simulink model "sim_all"  (R2020a)
settings: Solver=VariableStepAuto  StartTime=0.0  StopTime=2000  RelTol=1e-3
undefined symbols (not defined in the file or in its folder): a1, a2, alpha1, alpha2, cornerA, cornerB, cornerC, cornerD, ctrl_clockwise, ctrl_int_bound_or, ctrl_int_bound_pos, ctrl_k_or, ctrl_k_pos, ctrl_Ki_vel, ctrl_Kp_v_pos, ctrl_Kp_vel, ctrl_TAM, ctrl_Ts, ctrl_va_uncontrolled, ctrl_vel_uncontrolled, D, dead_zone_limit, depth, DiscIntNeverNeededParam, distanceFromWall, initInspectedSide, initPoint, mod_A, mod_Cd_F, mod_Cd_M, mod_eta_init, mod_g, mod_h0, mod_Ixx, mod_Iyy, mod_Izz, mod_Kp_dot, mod_lat0, mod_lon0, mod_m, mod_Mq_dot, mod_ni_init, mod_Nr_dot, mod_p1, mod_p2, mod_p3, mod_p4, mod_p5, mod_p6, mod_R, mod_Rm, mod_t1, mod_t2, mod_t3, mod_t4, mod_t5, mod_t6, mod_W, mod_Xu_dot, mod_Yv_dot ... (+53)
libraries: simulink x8, cstblocks x6, simulink_extras x1
(part 4 of 6)

== matlab function sim_all/Mission_supervisor_v3/Mission_Supervisor/Orientazione in profondità/MATLAB Function ==
  data: delta_current_or_prof output; delta_stato_or_prof output; Pos_d output size=3; Dpp_d output; Orp_d output; Pos_s input; Orp_s input; relativeDirection parameter; depth parameter; punto_iniz_patt input; error_flag input; soglia_orp parameter; soglia_SOS_pos parameter; SOS parameter; distanceFromWall parameter
function [delta_current_or_prof, delta_stato_or_prof, Pos_d, Dpp_d, Orp_d] = Orientazione_profondita(Pos_s, Orp_s, relativeDirection, depth, punto_iniz_patt, error_flag, soglia_orp, soglia_SOS_pos, SOS, distanceFromWall)

    disp("Orientazione in profondita");
    
    %% Unità di misura 
    
    % Pos_d, Pos_s, punto_iniz_patt, soglia_SOS_pos                        [deg, deg, m]
    % Orp_d, Orp_s, soglia_orp                                             [rad]
    % relativeDirection                                                    [deg]
    % Dpp_d, depth, distanceFromWall                                       [m]

    %% Inizializzazione variabili
    
    % Utilizzata per la permanenza nello stato corrente
    delta_stato_or_prof = 0;
    
    pronti = false;

    %% Preparazione dei riferimenti da fornire ai blocchi successivi
                
    % Posizione da mantenere
    Pos_d = [punto_iniz_patt(1); punto_iniz_patt(2); depth];
                                                                            %*****TEST******%
                                                                            %Pos_d = [43; 11; 0];
    
  
    % Orientazione da raggiungere
    Orp_d = deg2rad(relativeDirection);
    
    % Distanza dalla parete da mantenere
    Dpp_d = distanceFromWall;
    
    
    % Transizione di stato effettiva
    delta_current_or_prof = 104 - 103; 
    
    
    %% Verifiche
    
    % Verifica della corretta posizione
    if (abs(Pos_s(1) - Pos_d(1)) > soglia_SOS_pos(1) || ...
        abs(Pos_s(2) - Pos_d(2)) > soglia_SOS_pos(2) || ...
        abs(Pos_s(3) - Pos_d(3)) > soglia_SOS_pos(3))
    
        SOS = 1;
        disp("EMERGENZA:");
        
        if (abs(Pos_s(1) - Pos_d(1)) > soglia_SOS_pos(1))
            disp("Rilevato errore sulla posizione X");
        end
        if (abs(Pos_s(2) - Pos_d(2)) > soglia_SOS_pos(2))
            disp("Rilevato errore sulla posizione Y");
        end
        if (abs(Pos_s(3) - Pos_d(3)) > soglia_SOS_pos(3))
            disp("Rilevato errore sulla profondita Z");
        end
        
    end
    
    if error_flag == 1
        disp("EMERGENZA: errore segnalato dagli altri sottosistemi");
        SOS = 1;
    end
     
    % Si verifica di aver raggiunto l'orientazione desiderata
    if (SOS == 0 && ...
        abs(Orp_s - Orp_d) < soglia_orp)
    
        pronti = true;
    end
    
    %% Decisione dello stato successivo
    
    if pronti == true
        
        delta_stato_or_prof = 201 - 104; % Transizione eseguita correttamente
    end
    if SOS == 1
            
            delta_stato_or_prof = 301 - 104; % Transizione nello stato di emergenza
    end
    
    % Si rimane nello stato corrente
    

end

== matlab function sim_all/Mission_supervisor_v3/Mission_Supervisor/Frenata pattugliamento/MATLAB Function ==
  data: delta_current_fren_patt output; delta_stato_fren_patt output; contatore input; Pos_d output size=3; Dpp_d output; Dps_d output; Orp_d output; Pos_s input; Dpp_s input; Dps_s input; Orp_s input; distanceFromWall parameter; relativeDirection parameter; depth parameter; error_flag input; soglia_SOS_orp parameter; soglia_SOS_pos parameter; soglia_SOS_parete parameter; SOS parameter; soglia_parete parameter
function [delta_current_fren_patt, delta_stato_fren_patt, Pos_d, Dpp_d, Dps_d, Orp_d] = Frenata_pattugliamento(contatore, Pos_s, Dpp_s, Dps_s, Orp_s, distanceFromWall, relativeDirection, depth, error_flag, soglia_SOS_orp, soglia_SOS_pos, soglia_SOS_parete, SOS,soglia_parete)

    disp("Frenata (durante il pattugliamento)");
    
    %% Unità di misura 
    
    % Pos_d, Pos_s, soglia_SOS_pos                                                                 [deg, deg, m]
    % Orp_d, Orp_s, soglia_SOS_orp                                                                 [rad]
    % relativeDirection                                                                            [deg]
    % Dpp_d, Dps_d, Dpp_s, Dps_s, distanceFromWall, depth, soglia_SOS_parete, soglia_parete        [m]

    %% Inizializzazione variabili
   
    % Utilizzata per permanere nello stato corrente
    delta_stato_fren_patt = contatore;
    
    pronti = false;
    
    %% Preparazione dei riferimenti da fornire ai blocchi successivi
    
    % Profondità da mantenere
    Pos_d = [nan; nan; depth];
                                                                            %*****TEST******%
                                                                            %Pos_d = [nan; nan; 0];
    
    % Distanza dalla parete da mantenere
    Dpp_d = distanceFromWall;
    Dps_d = distanceFromWall;
    
    % Orientazione da mantenere
    Orp_d = deg2rad(relativeDirection);
    
    % Transizione di stato effettiva
    delta_current_fren_patt = 202 - 201 + contatore;  
    
    
    %% Verifiche
    
    % Verifica sulla corretta orientazione, profondità e distanza dalla parete pattugliata
    if (abs(Orp_s - Orp_d) > soglia_SOS_orp || ...
        abs(Dpp_s - Dpp_d) > soglia_SOS_parete || ...
        abs(Pos_s(3) - Pos_d(3)) > soglia_SOS_pos(3))
    
        SOS = 1;
        disp("EMERGENZA:");
        
        if (abs(Orp_s - Orp_d) > soglia_SOS_orp)
            disp("Rilevato errore sull'orientazione relativa");
        end
        
        if (abs(Dpp_s - Dpp_d) > soglia_SOS_parete)
            disp("Rilevato errore sulla distanza da parete");
        end
        
        if (abs(Pos_s(3) - Pos_d(3)) > soglia_SOS_pos(3))
            disp("Rilevato errore sulla profondita Z");
        end
        
    end
    
    if error_flag == 1
        disp("EMERGENZA: errore segnalato dagli altri sottosistemi");
        SOS = 1;
    end
     
                                                                            %*****TEST******%
                                                                            %test=0;
                                                                            %Serve per testare di rimanere 
                                                                            %in attesa in questo stato
                                                                            % if(contatore>2)
                                                                            %    test=100;
                                                                            % else
                                                                            %    test=0;
                                                                            % end

    % Si verifica di aver raggiunto la posizione desiderata in termini di 
    % distanza dalla parete successiva
    if (SOS == 0 && ...
        abs(Dps_s - Dps_d) < soglia_parete)
    
        pronti = true;
        
    end

    %% Decisione dello stato successivo
    
    if pronti == true
        
        delta_stato_fren_patt = 203 - 202 + contatore; % Transizione eseguita correttamente
    end
    if SOS == 1
            
            delta_stato_fren_patt = 301 - 202 + contatore; % Transizione nello stato di emergenza
    end
    % Si rimane nello stato corrente

end

== matlab function sim_all/Mission_supervisor_v3/Mission_Supervisor/Manovra/MATLAB Function ==
  data: delta_current_man output; delta_stato_man output; contatore output; contatore input; Pos_d output size=3; Dpp_d output; Dps_d output; Orp_d output; Pos_s input; Dpp_s input; Orp_s input; distanceFromWall parameter; relativeDirection parameter; depth parameter; error_flag input; soglia_orp parameter; soglia_SOS_parete parameter; soglia_SOS_pos parameter; SOS parameter; Dps_s input; alfa input; giro input; parete_attuale input
function [delta_current_man, delta_stato_man, contatore, Pos_d, Dpp_d, Dps_d, Orp_d] = Manovra(contatore, Pos_s, Dpp_s, Orp_s, distanceFromWall, relativeDirection, depth, error_flag, soglia_orp, soglia_SOS_parete, soglia_SOS_pos, SOS, Dps_s, alfa, giro, parete_attuale)

    disp("Manovra");
    
    %% Unità di misura 
     
    % Pos_d, Pos_s, soglia_SOS_pos                                                [deg,deg,m]
    % Orp_d, Orp_s, soglia_orp, alfa                                              [rad]
    % relativeDirection                                                           [deg]
    % Dpp_d, Dps_d, Dpp_s, Dps_s, distanceFromWall, depth, soglia_SOS_parete      [m]


    %% Inizializzazione variabili
    
    delta_stato_man = -2 * contatore;
    
    pronti = false;
    
    relativeDirection_rad = deg2rad(relativeDirection);
    
    % Si utilizza la variabile booleana giro, inizializzata nella matlab function "aggiornamento della parete"
    % per determinare il senso di pattugliamento
    if giro == 0 % orario
        inspectionDirection = "clockwise";
    else % antiorario
        inspectionDirection = "counterclockwise";
    end

    %% Preparazione dei riferimenti da fornire si blocchi successivi
          
    Pos_d = [nan; nan; depth];
                                                                            %*****TEST******%
                                                                            %Pos_d = [nan; nan; 0];
    % Distanza dalla parete da mantenere
    Dpp_d = distanceFromWall;
    Dps_d = distanceFromWall;
    
    % Orientazione relativa alla parete
    Orp_d = relativeDirection_rad;
    
    % In questo stato il riferimento di orientazione passato al controllo
    % si riferisce alla parete successiva. Questo rende necessario
    % l'introduzione della variabile "Orp_rif" utilizzata nelle condizioni
    % di switch poiché il valore di stima si riferisce ancora alla parete attuale.
    % I valori alfa corrispondono agli angoli interni ai corner del bacino.
    if (strcmp(inspectionDirection,'clockwise') == 1) % AB-BC-CD-DA
        
        if parete_attuale == 1 % pattugliamento AB, manovra in B
            Orp_rif = relativeDirection_rad + alfa(2); 
        elseif parete_attuale == 2 % pattugliamento BC, manovra in C
            Orp_rif = relativeDirection_rad + alfa(3);
        elseif parete_attuale == 3 % pattugliamento CD, manovra in D
            Orp_rif = relativeDirection_rad + alfa(4);
        else  % pattugliamento DA, manovra in A
            Orp_rif = relativeDirection_rad + alfa(1);
        end
        
    else % AB-DA-CD-BC
        
        if parete_attuale == 1 % pattugliamento AB, manovra in A
            Orp_rif = relativeDirection_rad - alfa(1);
        elseif parete_attuale == 2 % pattugliamento BC, manovra in B
            Orp_rif = relativeDirection_rad - alfa(2);
        elseif parete_attuale == 3 % pattugliamento CD, manovra in C
            Orp_rif = relativeDirection_rad - alfa(3);
        else % pattugliamento DA, manovra in D
            Orp_rif = relativeDirection_rad - alfa(4);
        end
    end
      
    % Transizione di stato effettiva
    delta_current_man = 203 - 202 + contatore;           
    
       
    %% Verifiche
    
    % Verifica di aver mantenuto la corretta profondità e distanza
    % dalle pareti considerate
    if (abs(Pos_s(3) - Pos_d(3)) > soglia_SOS_pos(3) || ...
       abs(Dpp_s - Dpp_d) > soglia_SOS_parete || ...
       abs(Dps_s - Dps_d) > soglia_SOS_parete)
    
        SOS = 1;
        disp("EMERGENZA:");
        
        if (abs(Pos_s(3) - Pos_d(3)) > soglia_SOS_pos(3))
            disp("Rilevato errore sulla profondita");
        end
        if (abs(Dpp_s - Dpp_d) > soglia_SOS_parete)
            disp("Rilevato errore sulla distanza da parete");
        end
        if (abs(Dps_s - Dps_d) > soglia_SOS_parete)
            disp("Rilevato errore sulla distanza da parete successiva");
        end
    end
    
                                                                            %*****TEST******%
                                                                            % if(contatore > 1)
                                                                            %     error_flag = 1;
                                                                            % end

     if error_flag == 1
        disp("EMERGENZA: errore segnalato dagli altri sottosistemi");
        SOS = 1;
     end
     
     
                                                                            %*****TEST******%
                                                                            %Serve per testare di rimanere 
                                                                            %in attesa in questo stato 
                                                                            %test = 0;
                                                                            %if(contatore > 2)%test
                                                                            %    test = 100;
                                                                            %else
                                                                            %    test = 0;
                                                                            %end
                                                                            
    % Si verifica di aver raggiunto l'orientazione desiderata 
    if (SOS == 0 && ...
        abs(Orp_s - Orp_rif) < soglia_orp)    
    
        pronti = true;
        
    end
    
    % La parete viene aggiornata soltanto
    % al termine della fase di manovra incrementando il contatore
    if pronti == true
         contatore = contatore + 1;
    end
    
     
    %% Decisione dello stato successivo
    
    if pronti == true
        if contatore < 4    % Non è ancora il pattugliamento dell'ultima parete 
            
            delta_stato_man = 201 - 203 - 2 * contatore +2;   % Si continua il pattugliamento delle pareti successive  
            
        else    % Completato il pattugliamento dell'ultima parete intera, si esce dal ciclo per
                % effettuare il pattugliamento parziale della parete
                % iniziale che era stata pattugliata solo per metà
                
            delta_stato_man = 204-203 - 2 * contatore +2;         
        end
    end
    
    if SOS == 1
            
            delta_stato_man = 301-203 + - 2 * contatore; %Transizione nello stato di emergenza
    end
        % Si rimane nello stato corrente

end

== matlab function sim_all/Mission_supervisor_v3/Mission_Supervisor/Completamento/MATLAB Function ==
  data: delta_current_comp output; parete input; delta_stato_comp output; Pos_d output size=3; Vel_d output; Dpp_d output; Orp_d output; Pos_s input; Vel_s input; Dpp_s input; Dps_s input; Orp_s input; depth parameter; speed parameter; distanceFromWall parameter; relativeDirection parameter; dps_fin input; error_flag input; soglia_SOS_vel parameter; soglia_parete_frenata parameter; soglia_SOS_orp parameter; soglia_SOS_pos parameter; soglia_SOS_parete parameter; SOS parameter; giro input
function [delta_current_comp, delta_stato_comp, Pos_d, Vel_d, Dpp_d, Orp_d] = Completamento(parete, Pos_s, Vel_s, Dpp_s, Dps_s, Orp_s, depth, speed, distanceFromWall, relativeDirection, dps_fin, error_flag, soglia_SOS_vel, soglia_parete_frenata, soglia_SOS_orp, soglia_SOS_pos, soglia_SOS_parete, SOS, giro)

    disp("Completamento del pattugliamento parziale della parete " + parete);
    
    %% Unità di misura 
    
    % Pos_d, Pos_s, soglia_SOS_pos                                                                              [deg, deg, m]
    % Orp_d, Orp_s, soglia_SOS_orp                                                                              [rad]
    % relativeDirection                                                                                         [deg]
    % Dpp_d, Dps_d, Dpp_s, Dps_s, dps_fin, distanceFromWall, depth, soglia_SOS_parete, soglia_parete_frenata    [m]
    % Vel_d, Vel_s, speed, soglia_SOS_vel                                                                       [m/s]

    %% Inizializzazione variabili
    
    % Utilizzata per permanere in questo stato e inizializzata a zero
    % perché fuori dal ciclo
    delta_stato_comp = 0; 
    
    pronti = false;
    
    
    %% Preparazione dei riferimenti da fornire ai blocchi successivi
    
    % Profondità da mantenere
    Pos_d = [nan; nan; depth];
                                                                            %*****TEST******%
                                                                            %Pos_d = [nan; nan; 0];
    
    % Velocità da raggiungere
    Vel_d = speed;              
                                                                            %*****TEST******%
                                                                            %Vel_d_vett = [0; 0; 0];

    % Distanza dalla parete da mantenere
    Dpp_d = distanceFromWall;
    
    % Orientazione da mantenere
    Orp_d = deg2rad(relativeDirection);
        
    % Transizione di stato effettiva
    delta_current_comp = 204 - 203;  
  
    %% Verifiche
    
    % Verifica sulla corretta profondità, orientazione, distanza dalla parete pattugliata 
    % e velocità
    if (abs(Pos_s(3) - Pos_d(3)) > soglia_SOS_pos(3) || ...
        abs(Orp_s - Orp_d) > soglia_SOS_orp || ...
        abs(Dpp_s - Dpp_d) > soglia_SOS_parete || ...
        norm(Vel_s) - Vel_d > soglia_SOS_vel)
    
        SOS = 1;
        disp("EMERGENZA:");
        
        if (abs(Orp_s - Orp_d) > soglia_SOS_orp)
            disp("Rilevato errore sull'orientazione relativa");
        end
        
        if (abs(Dpp_s - Dpp_d) > soglia_SOS_parete)
            disp("Rilevato errore sulla distanza da parete");
        end
        
        if (abs(Pos_s(3) - Pos_d(3)) > soglia_SOS_pos(3))
            disp("Rilevato errore sulla profondita Z");
        end
        
        if (norm(Vel_s) - Vel_d > soglia_SOS_vel)
            disp("Rilevato errore nella velocita");
        end

    end
    
                                                                            %*****TEST******%
                                                                            % if(contatore > 1)
                                                                            %     error_flag = 1;
                                                                            % end

     if error_flag == 1
        disp("EMERGENZA: errore segnalato dagli altri sottosistemi");
        SOS = 1;
     end
     
                                                                            %*****TEST******%
                                                                            %dps_fin = 4;

    % Si verifica di pattugliare alla velocità desiderata fino al punto di
    % frenata
    if (SOS == 0 && ...
        abs(Dps_s - (dps_fin + 3*speed)) < soglia_parete_frenata) % Analogo a quanto detto in "Pattugliamento"
    
        pronti = true;
        
    end
    
    %% Decisione dello stato successivo
    
    if pronti == true
        
        delta_stato_comp = 205 - 204; % Transizione eseguita correttamente
    end
    if SOS == 1
            
            delta_stato_comp = 301 - 204; % Transizione nello stato di emergenza
    end
  % Si rimane nello stato corrente.

end

== matlab function sim_all/Mission_supervisor_v3/Mission_Supervisor/Frenata in completamento/MATLAB Function ==
  data: delta_current_fren_comp output; delta_stato_fren_comp output; SOS_205 output; Pos_d output size=3; Dpp_d output; Dps_d output; Orp_d output; Pos_s input; Orp_s input; Dpp_s input; Dps_s input; depth parameter; distanceFromWall parameter; relativeDirection parameter; dps_fin input; error_flag input; soglia_SOS_pos parameter; soglia_SOS_parete parameter; soglia_SOS_orp parameter; soglia_parete parameter; SOS parameter
function [delta_current_fren_comp, delta_stato_fren_comp, SOS_205, Pos_d, Dpp_d, Dps_d, Orp_d] = Frenata_completamento(Pos_s, Orp_s, Dpp_s, Dps_s, depth, distanceFromWall, relativeDirection, dps_fin, error_flag, soglia_SOS_pos, soglia_SOS_parete, soglia_SOS_orp, soglia_parete, SOS)

    disp("Frenata (durante il completamento del pattugliamento parziale)");
    
    %% Unità di misura 
    
    % Pos_d, Pos_s, soglia_SOS_pos                                                                      [deg, deg, m]
    % Orp_d, Orp_s, soglia_SOS_orp                                                                      [rad]
    % relativeDirection                                                                                 [deg]
    % Dpp_d, Dps_d, Dpp_s, Dps_s, dps_fin, distanceFromWall, depth, soglia_SOS_parete, soglia_parete    [m]
    
    %% Inizializzazione variabili
    
    delta_stato_fren_comp = 0;
    
    pronti = false;
    

    %% Preparazione dei riferimenti da fornire si blocchi successivi
    
    % Profondità da mantenere
    Pos_d = [nan; nan; depth];
                                                                            %*****TEST******%
                                                                            %Pos_d = [nan;nan;0];
    % Distanza dalla parete da mantenere
    Dpp_d = distanceFromWall;
    Dps_d = dps_fin;
    
    % Orientazione da mantenere
    Orp_d = deg2rad(relativeDirection);
    
    % Transizione di stato effettiva
    delta_current_fren_comp = 205 - 204;  
    
       
    %% Verifiche

    % Si verifica la corretta orientazione, profondità e distanza dalla parete di pattugliamento 
    if (abs(Pos_s(3) - Pos_d(3)) > soglia_SOS_pos(3) || ...
        abs(Orp_s - Orp_d) > soglia_SOS_orp || ...
        abs(Dpp_s - Dpp_d) > soglia_SOS_parete)
    
        SOS = 1;
        pronti = true;
        disp("EMERGENZA:");
        
        if (abs(Pos_s(3) - Pos_d(3)) > soglia_SOS_pos(3))
            disp("Rilevato errore sulla profondita Z");
        end
        
        if (abs(Orp_s - Orp_d) > soglia_SOS_orp)
            disp("Rilevato errore sull'orientazione relativa");
        end
        
        if (abs(Dpp_s - Dpp_d) > soglia_SOS_parete)
            disp("Rilevato errore sulla distanza da parete");
        end
    end
    
    if error_flag == 1
        disp("EMERGENZA: errore segnalato dagli altri sottosistemi");
        SOS = 1;
    end
 
    SOS_205 = SOS;                                                                     %*****TEST******%
                                                                            %dps_fin = 8;

    % Si verifica di aver raggiunto la posizione desiderata di fine pattugliamento
    if (SOS==0 && ...
        abs(Dps_s - dps_fin) < soglia_parete) 
        pronti = true;
        
    end
    
    %% Decisione dello stato successivo
    
    if (pronti == true || SOS == 1)
        
        delta_stato_fren_comp = 301 - 205; % Transizione di stato
    end
    % Si rimane nello stato corrente
    

end

== matlab function sim_all/Mission_supervisor_v3/Mission_Supervisor/Orientazione in superficie/MATLAB Function ==
  data: delta_current_or_sup output; delta_stato_or_sup output; Or_in input; error_flag input; punto_iniz_patt input; SOS parameter; Pos_d output size=3; Or_d output size=3; soglia_SOS_pos parameter; soglia_or parameter; Pos_s input; Or_s input; soglia_SOS_or parameter
function [delta_current_or_sup, delta_stato_or_sup, Pos_d, Or_d] = Orientazioneinsuperficie(Or_in, error_flag, punto_iniz_patt, SOS, soglia_SOS_pos, soglia_or, Pos_s, Or_s, soglia_SOS_or)

    disp("Orientazione in superficie");
    
    %% Unità di misura 
    
    % Pos_d, Pos_s, soglia_SOS_pos, punto_iniz_patt                             [deg,deg,m]
    % Or_d, Or_in, Or_s, soglia_SOS_or, soglia_or                               [deg,deg,deg]

    %% Inizializzazione variabili
    
    delta_stato_or_sup = 0;
    
    pronti = false; 

    %% Preparazione dei riferimenti da fornire ai blocchi successivi
  
    % Posizione da mantenere
    Pos_d = punto_iniz_patt; 
                                                                            %*****TEST******%
                                                                            %Pos_d = [43; 11; 0];  
    % Orientazione desiderata e necessaria per raggiungere
    % il punto di rientro
    Or_d = Or_in;
                                                                            %*****TEST******%
                                                                            %Or_d = [1; 1; 1];
  
    % Transizione di stato effettiva
    delta_current_or_sup = 302 - 301;
   
    
    %% Verifiche 
    
    % Verifica della posizione e dell'orientazione
   if (abs(Pos_s(1) - Pos_d(1)) > soglia_SOS_pos(1) || ...
       abs(Pos_s(2) - Pos_d(2)) > soglia_SOS_pos(2) || ...
       abs(Pos_s(3) - Pos_d(3)) > soglia_SOS_pos(3) || ...
       abs(Or_s(1) - Or_d(1)) > soglia_SOS_or(1) || ...
       abs(Or_s(2) - Or_d(2)) > soglia_SOS_or(2))
    
        SOS = 1;
        disp("EMERGENZA:");
        
        
        if (abs(Pos_s(1) - Pos_d(1)) > soglia_SOS_pos(1))
            disp("Rilevato errore sulla posizione X");
        end
        if (abs(Pos_s(2) - Pos_d(2)) > soglia_SOS_pos(2))
            disp("Rilevato errore sulla posizione Y");
        end
        if (abs(Pos_s(3) - Pos_d(3)) > soglia_SOS_pos(3))
            disp("Rilevato errore sulla profondita Z");
        end
        if (abs(Or_s(1) - Or_d(1)) > soglia_SOS_or(1))
            disp("Rilevato errore sulla rotazione di roll");
        end
        if (abs(Or_s(2) - Or_d(2)) > soglia_SOS_or(2))
            disp("Rilevato errore sulla rotazione di pitch");
        end

    end
    
    if error_flag == 1
        disp("EMERGENZA: errore segnalato dagli altri sottosistemi");
        SOS = 1;
    end
    
    % Si verifica di aver raggiunto l'orientazione desiderata
    if  (SOS == 0 && ...
         abs(Or_s(3) - Or_d(3)) < soglia_or(3))
    
        pronti = true;
        
    end
    
%% Decisione dello stato successivo
    
    if pronti == true
       
        delta_stato_or_sup = 303 - 302; % Transizione eseguita correttamente
    end
    
    if SOS == 1
            
            delta_stato_or_sup = 304 - 302; % Transizione nello stato di emergenza
    end

    % Si rimane nello stato corrente
end

== matlab function sim_all/Mission_supervisor_v3/Mission_Supervisor/Pattugliamento/MATLAB Function ==
  data: parete input; contatore input; delta_current_patt output; Pos_s input; Dpp_s input; Dps_s input; delta_stato_patt output; Pos_d output size=3; Vel_d output; Dpp_d output; Orp_d output; Orp_s input; Vel_s input; depth parameter; speed parameter; distanceFromWall parameter; relativeDirection parameter; soglia_parete_frenata parameter; soglia_SOS_orp parameter; soglia_SOS_parete parameter; soglia_SOS_pos parameter; error_flag input; SOS parameter; soglia_SOS_vel parameter; giro input
function [delta_current_patt, delta_stato_patt, Pos_d, Vel_d, Dpp_d, Orp_d] = Pattugliamento(parete, contatore, Pos_s, Dpp_s, Dps_s, Orp_s, Vel_s, depth, speed, distanceFromWall, relativeDirection, soglia_parete_frenata, soglia_SOS_orp, soglia_SOS_parete, soglia_SOS_pos, error_flag, SOS, soglia_SOS_vel, giro)
    
    % In base al valore del contatore un display mostra il tipo di pattugliamento (parziale o completo)
    if contatore == 0
        disp("Pattugliamento parziale parete " + parete);
    else
        disp("Pattugliamento parete " + parete);
    end 
    
    %% Unità di misura 
    
    % Pos_d, Pos_s, soglia_SOS_pos                                                        [deg, deg, m]
    % Orp_d, Orp_s, soglia_SOS_orp                                                        [rad]
    % relativeDirection                                                                   [deg]
    % Dpp_d,Dpp_s, depth, distanceFromWall, soglia_parete_frenata, soglia_SOS_parete      [m]
    % Vel_d, Vel_s, speed, soglia_SOS_vel                                                 [m/s]

    
    %% Inizializzazione variabili
    
    % Si attribuisce alla variabile delta_stato_patt il valore contatore per  
    % tenere traccia delle transizioni effettuate durante il ciclo di
    % pattugliamento. Questo deve essere fatto perché i valori delta_stato
    % rimangono attivi una volta inizializzati nel ciclo.
    delta_stato_patt = contatore;
    
    pronti = false;
    
    %% Preparazione dei riferimenti da fornire ai blocchi successivi
    
    % Profondità da mantenere
    Pos_d = [nan; nan; depth];
                                                                            %*****TEST******%
                                                                            %Pos_d = [nan;nan;0];
    
    % Velocità da raggiungere
    Vel_d = speed;             

    % Distanza dalla parete da mantenere
    Dpp_d = distanceFromWall;
    
    % Orientazione da mantenere
    Orp_d = deg2rad(relativeDirection);
    
    
    % Transizione di stato effettiva a seconda che si arrivi da
    % "Orientazione in profondità" o da "Manovra"
    delta_current_patt = 201-104;   
   
    if contatore>0
        delta_current_patt = 201 - 104 - (2*contatore); 
    end
       
    %% Verifiche
    
    %Verifica sull'orientazione, sulla velocità, sulla profondità e sulla
    %distanza dalla parete pattugliata
    if (abs(Pos_s(3) - Pos_d(3)) > soglia_SOS_pos(3) || ...
        abs(Orp_s - Orp_d) > soglia_SOS_orp || ...
        norm(Vel_s) - Vel_d > soglia_SOS_vel || ...
        abs(Dpp_s - Dpp_d) > soglia_SOS_parete)
 
        SOS = 1;
        disp("EMERGENZA:");
        
        if (abs(Orp_s-Orp_d) > soglia_SOS_orp)
            disp("Rilevato errore sull'orientazione relativa");
        end
        if (abs(Dpp_s - Dpp_d) > soglia_SOS_parete)
            disp("Rilevato errore sulla distanza da parete");
        end
        if (abs(Pos_s(3) - Pos_d(3)) > soglia_SOS_pos(3))
            disp("Rilevato errore sulla profondita");
        end
        if (norm(Vel_s) - Vel_d > soglia_SOS_vel)
            disp("Rilevato errore sulla velocita");
        end

    end
%                                                                             %*****TEST******%
%                                                                             if(contatore>1)
%                                                                                 error_flag=1;
%                                                                             end

     if error_flag == 1
        disp("EMERGENZA: errore segnalato dagli altri moduli");
        SOS = 1;
     end
                                                                            %*****TEST******%
                                                                            %Serve per testare di rimanere 
                                                                            %in attesa in questo stato 
                                                                            %test=0;
%                                                                             if(contatore>1)%test
%                                                                                test=100;
%                                                                             else
%                                                                                test=0;
%                                                                             end
    
    % Si verifica di pattugliare fino al punto di frenata calcolata
    % considerando un tempo di frenata di tre secondi
    if (SOS == 0 && ...
        abs(Dps_s - (distanceFromWall + 3*speed)) < soglia_parete_frenata) 

        
        pronti = true;
        
    end
    
    %% Decisione dello stato successivo
    
    if pronti == true

        delta_stato_patt = 202 - 201 + contatore; %Transizione eseguita correttamente
    end
    if SOS == 1
            
            delta_stato_patt = 301 - 201 + contatore; %Transizione nello stato di emergenza
    end
% Si rimane nello stato corrente

end

== matlab function sim_all/Mission_supervisor_v3/Mission_Supervisor/Fine missione/MATLAB Function ==
  data: delta_current_end output; stato input
function delta_current_end  = Fine_missione(stato)

    disp("Fine missione");
    
    
    
    %% Transizione di stato effettiva 
    delta_current_end = 304 - stato;  
    
    % La missione è conclusa e la simulazione termina.

end

== matlab function sim_all/Mission_supervisor_v3/Mission_Supervisor/Posizionamento/MATLAB Function ==
  data: delta_current_posiz output; delta_stato_posiz output; Pos_d output size=3; Or_d output size=3; Pos_s input; Or_s input; punto_iniziale input; Or_in input; error_flag input; soglia_pos parameter; soglia_SOS_or parameter; SOS parameter; soglia_SOS_pos parameter
function [delta_current_posiz, delta_stato_posiz, Pos_d, Or_d] = Posizionamento(Pos_s, Or_s, punto_iniziale, Or_in, error_flag, soglia_pos, soglia_SOS_or, SOS, soglia_SOS_pos)

    disp("Posizionamento");
    
    %% Unità di misura 
    
    % Pos_d, Pos_s, punto_iniziale, soglia_pos, soglia_SOS_pos             [deg, deg, m]
    % Or_d, Or_s, Or_in, soglia_SOS_or                                     [rad, rad, rad]

    %% Inizializzazione variabili
    
    % Mantenimento dello stato_interno al valore
    % desiderato durante la permanenza del sistema nello stato corrente.
    delta_stato_posiz = 0;
    
    pronti = false;
   
    %% Preparazione dei riferimenti da fornire ai blocchi successivi
    
    % Posizione da raggiungere
    Pos_d = punto_iniziale;                                                %*****TEST******%
                                                                            %Pos_d = [43; 11; 0];
     
   
    % Orientazione da mantenere
    Or_d = Or_in;
    
    % Transizione di stato effettiva
    delta_current_posiz = 102 - 101;  
       
    
    %% Verifiche
    
     % Verifica della corretta orientazione e profondità
     
    if (abs(Or_s(1) - Or_d(1)) > soglia_SOS_or(1) || ...
        abs(Or_s(2) - Or_d(2)) > soglia_SOS_or(2) || ...
        abs(Or_s(3) - Or_d(3)) > soglia_SOS_or(3) || ...
        abs(Pos_s(3) - Pos_d(3)) > soglia_SOS_pos(3))
    
        SOS = 1;
        disp("EMERGENZA:");       
        
        if (abs(Or_s(1) - Or_d(1)) > soglia_SOS_or(1))
            disp("Rilevato errore sulla rotazione di roll");
        end
        
        if (abs(Or_s(2) - Or_d(2)) > soglia_SOS_or(2))
            disp("Rilevato errore sulla rotazione di pitch");
        end
        
        if (abs(Or_s(3) - Or_d(3)) > soglia_SOS_or(3))
            disp("Rilevato errore sulla rotazione di yaw");
        end
       
        if (abs(Pos_s(3) - Pos_d(3)) > soglia_SOS_pos(3))
            disp("Rilevato errore sulla posizione lungo z");
        end
        
    end
    
    if error_flag == 1
        disp("EMERGENZA: errore segnalato dagli altri sottosistemi");
        SOS = 1;
    end
    
    % Si verifica di aver raggiunto la posizione desiderata
    if (SOS == 0 && ...
        abs(Pos_s(1) - Pos_d(1)) < soglia_pos(1) && ...
        abs(Pos_s(2) - Pos_d(2)) < soglia_pos(2))
    
        pronti = true;
        
    end

    %% Decisione dello stato successivo
     
    if pronti == true
        
        delta_stato_posiz = 103 - 102; % Transizione eseguita correttamente
    end
    if SOS == 1
            
            delta_stato_posiz = 304 - 102; % Transizione nello stato di emergenza
    end
    % Si rimane nello stato corrente

end

== matlab function sim_all/Mission_supervisor_v3/Mission_Supervisor/Rientro/MATLAB Function ==
  data: delta_current_rient output; delta_stato_rient output; Pos_d output size=3; Pos_s input; initPoint parameter; Or_in input; Or_d output size=3; soglia_pos parameter; SOS parameter; error_flag input; Dps_s input; Dpp_s input; soglia_SOS_collisione parameter; soglia_SOS_or parameter; soglia_SOS_pos parameter; Or_s input
function [delta_current_rient, delta_stato_rient, Pos_d, Or_d] = Rientro(Pos_s, initPoint, Or_in, soglia_pos, SOS, error_flag, Dps_s, Dpp_s, soglia_SOS_collisione, soglia_SOS_or, soglia_SOS_pos, Or_s)

    disp("Rientro");
    
    %% Unità di misura 
    
    % Pos_d, Pos_s, soglia_pos, initPoint, soglia_SOS_pos                    [deg,deg,m]
    % Or_d, Or_in, Or_s, soglia_SOS_or                                       [deg,deg,deg]
    % Dps_s, Dpp_s, soglia_SOS_collisione_s                                  [m]

    %% Inizializzazione variabili
    
    delta_stato_rient = 0;
    
    pronti = false;
    
    %% Preparazione dei riferimenti da fornire ai blocchi successivi
      
    % Posizione da raggiungere
    Pos_d = initPoint;
    
    % Orientazione da mantenere
    Or_d = Or_in;
    
    % Transizione di stato effettiva
    delta_current_rient = 303 - 302; 
       
    %% Verifiche
    
    % Verifica sulla profondità, sull'orientazione e sull'assenza di collisioni
    if (Dpp_s  < soglia_SOS_collisione || ... 
        Dps_s < soglia_SOS_collisione || ...
        abs(Or_s(1) - Or_d(1)) > soglia_SOS_or(1) || ...
        abs(Or_s(2) - Or_d(2)) > soglia_SOS_or(2) || ...
        abs(Or_s(3) - Or_d(3)) > soglia_SOS_or(3) || ...
        abs(Pos_s(3) - Pos_d(3)) > soglia_SOS_pos(3))
            
    
        SOS = 1;
        disp("EMERGENZA:");  
 

        if (Dpp_s < soglia_SOS_collisione || ... 
            Dps_s < soglia_SOS_collisione)
            disp("Pericolo collisione");
        end
        
        if (abs(Or_s(1) - Or_d(1)) > soglia_SOS_or(1))
            disp("Rilevato errore sulla rotazione di roll");
        end
        
        if (abs(Or_s(2) - Or_d(2)) > soglia_SOS_or(2))
            disp("Rilevato errore sulla rotazione di pitch");
        end
        
        if (abs(Or_s(3) - Or_d(3)) > soglia_SOS_or(3))
            disp("Rilevato errore sulla rotazione di yaw");
        end
     
        if (abs(Pos_s(3) - Pos_d(3)) > soglia_SOS_pos(3))
            disp("Rilevato errore sulla posizione lungo z");
        end
    
    end
    
    if error_flag == 1
        
        disp("EMERGENZA: errore segnalato dagli altri sottosistemi");
        SOS = 1;
        
    end
   
    % Si verifica di aver raggiunto la posizione desiderata
    if (SOS == 0 && ...
        abs(Pos_s(1) - Pos_d(1)) < soglia_pos(1) && ...
        abs(Pos_s(2) - Pos_d(2)) < soglia_pos(2))
    
        pronti = true;
        
    end
    

    
   %% Decisione dello stato successivo
    
   % Si effettua la transizione nello stato successivo indipendentemente
   % dal verificarsi di una emergenza
    if (pronti == true || SOS == 1)

        delta_stato_rient = 304 - 303;
    end
    % Si rimane nello stato corrente

end

== matlab function sim_all/Sensors/MATLAB Function ==
  data: u input; y output
function y = fcn(u)
 if u(3)==0
     u(1)=NaN;
     u(2)=NaN; 
 end
y = u;

== matlab function sim_all/Controller_mk4_v3/C_or/C_or_X ==
  data: err_int output; ang input; vel output; k input; ctrl_va_uncontrolled parameter; ctrl_int_bound_or parameter
%% Azione proporzionale
function [err_int, vel] = fcn(ang, k, ctrl_va_uncontrolled, ctrl_int_bound_or)
    v = 0;
    err_int = 0;
    va_des = ctrl_va_uncontrolled;  % velocità impostata prima della fase di frenata
    brake_dist = (1/k)*va_des;      % distanza in cui dobbiamo iniziare a frenare
    if ang >= brake_dist            % al di fuori dello spazio di frenata
        v = va_des;
    end
    if ang <= -brake_dist           % al di fuori dello spazio di frenata in negativo
        v = -va_des;
    end
    if  abs(ang) < brake_dist       % proporzionale se entro la distanza di frenata
        v = k*ang;
    end
    vel = v;
    if abs(ang) < ctrl_int_bound_or    % per il regime può essere utile una azione integrale
        err_int = ang;                 % err_int va ad un integratore
    end
end

== matlab function sim_all/Controller_mk4_v3/C_or/C_or_Y ==
  data: err_int output; ang input; vel output; k input; ctrl_va_uncontrolled parameter; ctrl_int_bound_or parameter
%% Azione proporzionale
function [err_int, vel] = fcn(ang, k, ctrl_va_uncontrolled, ctrl_int_bound_or)
    v = 0;
    err_int = 0;
    va_des = ctrl_va_uncontrolled;  % velocità impostata prima della fase di frenata
    brake_dist = (1/k)*va_des;      % distanza in cui dobbiamo iniziare a frenare
    if ang >= brake_dist            % al di fuori dello spazio di frenata
        v = va_des;
    end
    if ang <= -brake_dist           % al di fuori dello spazio di frenata in negativo
        v = -va_des;
    end
    if  abs(ang) < brake_dist       % proporzionale se entro la distanza di frenata
        v = k*ang;
    end
    vel = v;
    if abs(ang) < ctrl_int_bound_or    % per il regime può essere utile una azione integrale
        err_int = ang;                 % err_int va ad un integratore
    end
end

== matlab function sim_all/Controller_mk4_v3/C_or/C_or_Z ==
  data: err_int output; ang input; vel output; k input; ctrl_va_uncontrolled parameter; ctrl_int_bound_or parameter
%% Azione proporzionale
function [err_int, vel] = fcn(ang, k, ctrl_va_uncontrolled, ctrl_int_bound_or)
    v = 0;
    err_int = 0;
    va_des = ctrl_va_uncontrolled;  % velocità impostata prima della fase di frenata
    brake_dist = (1/k)*va_des;      % distanza in cui dobbiamo iniziare a frenare
    if ang >= brake_dist            % al di fuori dello spazio di frenata
        v = va_des;
    end
    if ang <= -brake_dist           % al di fuori dello spazio di frenata in negativo
        v = -va_des;
    end
    if  abs(ang) < brake_dist       % proporzionale se entro la distanza di frenata
        v = k*ang;
    end
    vel = v;
    if abs(ang) < ctrl_int_bound_or    % per il regime può essere utile una azione integrale
        err_int = ang;                 % err_int va ad un integratore
    end
end

== matlab function sim_all/Controller_mk4_v3/C_pos/C_pos_X ==
  data: err_int output; pos input; vel output; k input; ctrl_vel_uncontrolled parameter; ctrl_int_bound_pos parameter
%% Azione proporzionale
function [err_int, vel] = fcn(pos, k, ctrl_vel_uncontrolled, ctrl_int_bound_pos)
    v = 0;
    err_int = 0;
    vel_des = ctrl_vel_uncontrolled;    % velocità impostata se 'lontani'
    brake_dist = 1/k*vel_des;           % distanza di frenata
    if pos >= brake_dist                % se ho spazio per frenare mantengo la velocità
        v = vel_des;
    end
    if pos <= -brake_dist               % lontani in direzione negativa
        v = -vel_des;
    end
    if  abs(pos) < brake_dist           % se è vicino il proporzionale gestisce la frenata
        v = k*pos;
    end
    vel = v;
    if abs(pos) < ctrl_int_bound_pos    % per il regime può essere utile una azione integrale
        err_int = pos;                  % err_int va ad un integratore
    end

== matlab function sim_all/Controller_mk4_v3/C_pos/C_pos_Z ==
  data: err_int output; pos input; vel output; k input; ctrl_vel_uncontrolled parameter; ctrl_int_bound_pos parameter
%% Azione proporzionale
function [err_int, vel] = fcn(pos, k, ctrl_vel_uncontrolled, ctrl_int_bound_pos)
    v = 0;
    err_int = 0;
    vel_des = ctrl_vel_uncontrolled;    % velocità impostata se 'lontani'
    brake_dist = 1/k*vel_des;           % distanza di frenata
    if pos >= brake_dist                % se ho spazio per frenare mantengo la velocità
        v = vel_des;
    end
    if pos <= -brake_dist               % lontani in direzione negativa
        v = -vel_des;
    end
    if  abs(pos) < brake_dist           % se è vicino il proporzionale gestisce la frenata
        v = k*pos;
    end
    vel = v;
    if abs(pos) < ctrl_int_bound_pos    % per il regime può essere utile una azione integrale
        err_int = pos;                  % err_int va ad un integratore
    end

== matlab function sim_all/Controller_mk4_v3/InputOr_Organizer/diff_or ==
  data: or_d input; err_or output; or_s input
%% Calcolo errore
function err_or = fcn(or_d, or_s)
coder.extrinsic('wrapToPi');
err_or = zeros(3,1);
err_or = wrapToPi(or_d - or_s);    % rimane compreso tra -pi e +pi
end

== matlab function sim_all/Controller_mk4_v3/InputPos_Organizer/Ned2Body1 ==
  data: x_n input size=[3 1]; x_b output size=[3 1]; or input
%% Da NED a BODY
function x_b = ned2body(x_n,or)
C=zeros(3,3);
C=Cx(or(1))'*Cy(or(2))'*Cz(or(3))';
x_b = C'*x_n;
end

== matlab function sim_all/Controller_mk4_v3/InputPos_Organizer/Ned2Body2 ==
  data: x_n input size=[3 1]; x_b output size=[3 1]; or input
%% Da NED a BODY
function x_b = ned2body(x_n,or)
C=zeros(3,3);
C=Cx(or(1))'*Cy(or(2))'*Cz(or(3))';
x_b = C'*x_n;
end

== matlab function sim_all/Navigation/Extended Kalman Filter/MATLAB Function5 ==
  data: u input; dev_standard_x output; dev_standard_y output; dev_standard_z output
function [dev_standard_x,dev_standard_y,dev_standard_z] = fcn(u) 
    
    dev_standard_x = sqrt(u(1,1));
    dev_standard_y = sqrt(u(2,2));
    dev_standard_z = sqrt(u(3,3));
end

== matlab function sim_all/Controller_mk4_v3/InputPos_Organizer/Ned2Body3 ==
  data: x_n input size=[3 1]; x_b output size=[3 1]; or input
%% Da NED a BODY
function x_b = ned2body(x_n,or)
C=zeros(3,3);
C=Cx(or(1))'*Cy(or(2))'*Cz(or(3))';
x_b = C'*x_n;
end

== matlab function sim_all/Controller_mk4_v3/InputPos_Organizer/Ned2Body4 ==
  data: x_n input size=[3 1]; x_b output size=[3 1]; or input
%% Da NED a BODY
function x_b = ned2body(x_n,or)
C=zeros(3,3);
C=Cx(or(1))'*Cy(or(2))'*Cz(or(3))';
x_b = C'*x_n;
end

== matlab function sim_all/Controller_mk4_v3/InputPos_Organizer/brake_trigger ==
  data: state input; trigg_brake output
%% Restituisce 0 se in frenata
% In frenata vengono controllate sia dpp che dps
function trigg_brake = fcn(state)
tmp = 0;
switch state
    case 100            % fermo in superficie
        tmp = 1;
    case 101            % orientazione verso parete di inizio in superficie
        tmp = 1;
    case 102            % posizionamento in superficie
        tmp = 1;   
    case 103            % immersione
        tmp = 1;
    case 104            % orientazione in profondità
        tmp = 1;
    case 201            % pattugliamento
        tmp = 1;
    case 202            % frenata
        tmp = 0;
    case 203            % manovra di cambio parete
        tmp = 0;
    case 204            % competamento del pattugliamento della parete iniziale
        tmp = 1;
    case 205            % frenata a metà parete
        tmp = 0;
    case 301            % risalita
        tmp = 0;
    case 302            % orientazione in superficie
        tmp = 1;
    case 303            % rientro, ritorno al punto iniziale in superficie
        tmp = 1;
    case 304            % fine missione, tutto spento
        tmp = 1;
end
trigg_brake = tmp;
end

== matlab function sim_all/Controller_mk4_v3/InputVel_Organizer/Ned2Body4 ==
  data: x_n input size=[3 1]; x_b output size=[3 1]; or input
%% Da NED a BODY
function x_b = ned2body(x_n,or)
C=zeros(3,3);
C=Cx(or(1))'*Cy(or(2))'*Cz(or(3))';
x_b = C'*x_n;
end
